simulink model "dsPIC33CK256MP508_MCLV2_QEI_Generator"  (R2022a)
settings: Solver=FixedStepDiscrete  StartTime=0.0  StopTime=12  FixedStep=.00005  RelTol=1e-3  EnableMultiTasking=on
PostLoadFcn:
  | dsPIC33CK256MP508_MCLV2_Generator_data;
InitFcn:
  | dsPIC33CK256MP508_MCLV2_Generator_data;
values from neighbouring files (symbols this model uses):
  dataType = fixdt(1,16,14)    [dsPIC33CK256MP508_MCLV2_Generator_data.m]    (also in dsPIC33CK256MP508_MCLV2_SMO_data.m; mcb_pmsm_foc_qep_dsPIC33_data.m)
  PI_params = mcb.internal.SetControllerParameters(pmsm,inverter,PU_System,T_pwm,2*Ts,Ts_speed)    [dsPIC33CK256MP508_MCLV2_Generator_data.m]    (also in dsPIC33CK256MP508_MCLV2_SMO_data.m = mcb.internal.SetControllerParameters(pmsm,inverter,PU_System; mcb_pmsm_foc_qep_dsPIC33_data.m)
  PU_System = mcb_SetPUSystem(pmsm,inverter)    [dsPIC33CK256MP508_MCLV2_Generator_data.m]    (also in dsPIC33CK256MP508_MCLV2_SMO_data.m; mcb_pmsm_foc_qep_dsPIC33_data.m)
  PWM_frequency = 20e3    (= 20000)    [dsPIC33CK256MP508_MCLV2_Generator_data.m]    (also in dsPIC33CK256MP508_MCLV2_SMO_data.m; mcb_pmsm_foc_qep_dsPIC33_data.m)
  Ts = T_pwm    (= 5e-05)    [dsPIC33CK256MP508_MCLV2_Generator_data.m]    (also in dsPIC33CK256MP508_MCLV2_SMO_data.m; mcb_pmsm_foc_qep_dsPIC33_data.m)
  Ts_speed = 10*Ts    (= 0.0005)    [dsPIC33CK256MP508_MCLV2_Generator_data.m]    (also in dsPIC33CK256MP508_MCLV2_SMO_data.m = 0.0015; mcb_pmsm_foc_qep_dsPIC33_data.m)
undefined symbols (not defined in the file or in its folder): A4, AN1, B0, B15, B2, B9, C9, D1, D2, D6, inverter, MaxPer, P20, P32, P41, P47, P57, P65, P66, P70, Pin, pmsm, PWM1max, Resol, s, us
libraries: MCHP_Blockset x14, simulink x10, mcbcontrolslib x8, slpidlib x2, mcbpositiondecoderlib x2
(part 2 of 2)

== system dsPIC33CK256MP508_MCLV2_QEI_Generator/MOTOR Cmd ==
  PWM (abc) : Inport
  Dead time Compensation : Bias  Bias=round( (2e-6/5e-5) *PWM1max )  SaturateOnIntegerOverflow=off
  Demux : Demux  Outputs=3
  PWM_HS_FEP : MCHP_Blockset/PWM IO/PWM_HS_FEP  Priority=-2000  PWMx_MODSEL=Center Aligned  PWMx_CLKSEL=no scaling  PWM_ClockResolution_DIVSEL=Dynamic Options  PWM_ClockResolution_DIVSEL_TXT=auto  PWM_ClockResolution_FSCL=Dynamic Options  PWM_ClockResolution_FSCL_TXT=auto - no jitter  PWM_ClockResolution_NoScaling=Dynamic Options  PWM_ClockResolution_NoScaling_TXT="Resol: 0.005(us)  -  MaxPer: 0.000328(s)"  MaxPeriod_s=50e-6  InitPeriode_s=50e-6  InitDutyCycleP_s=2e-6  InitDutyCycleS_s=10e-6  InitPhase_s=-1  evalin_ws=PWM1max=MCHP_Fun.Hex2num('40B3880000000000');PWM2max=MCHP_Fun.Hex2num('40B3880000000000');PWM3max=MCHP_Fun.Hex2num('40B3880000000000');  SampleTime=-1  S_INPUT=[-1]  S_INPUT_Size=[3]  S_OUTPUT=[]  S_OUTPUT_Size=[]  S_ListCustomDatatype=S.S_ListCustomDatatype={};  MCHP_USER_INTERRUPTS=0  MCHP_PORT={PWMH1 }{PWMH1}32:4:B14;{PWMH2 }{PWMH2}32:4:B12;{PWMH3 }{PWMH3}32:4:B10;{PWML1}{PWML1}32:4:B15;{PWML2}{PWML2}32:4:B13;{PWML3}{PWML3}32:4:B11;  MCHP_MASTERLINK=dsPIC33CK256MP508_MCLV2_QEI_Generator/Hardware Init/Microchip Master  MCHP_CRC=4854455  PWMx_PMOD=Complementary  PWM1_HL=PWMxH & PWMxL output enabled  PWM1_swap=off  PWM1H_pol=off  PWM1L_pol=off  PWM2_HL=PWMxH & PWMxL output enabled  PWM2_swap=off  PWM2H_pol=off  PWM2L_pol=off  PWM3_HL=PWMxH & PWMxL output enabled  PWM3_swap=off  PWM3H_pol=off  PWM3L_pol=off  PWM4_HL=not used  PWM4_swap=off  PWM4H_pol=off  PWM4L_pol=off  PWM5_HL=not used  PWM5_swap=off  PWM5H_pol=off  PWM5L_pol=off  PWM6_HL=not used  PWM6_swap=off  PWM6H_pol=off  PWM6L_pol=off  PWM7_HL=not used  PWM7_swap=off  PWM7H_pol=off  PWM7L_pol=off  PWM8_HL=not used  PWM8_swap=off  PWM8H_pol=off  PWM8L_pol=off  PWM9_HL=not used  PWM9_swap=off  PWM9H_pol=off  PWM9L_pol=off  PWM10_HL=not used  PWM10_swap=off  PWM10H_pol=off  PWM10L_pol=off  PWM11_HL=not used  PWM11_swap=off  PWM11H_pol=off  PWM11L_pol=off  PWM12_HL=not used  PWM12_swap=off  PWM12H_pol=off  PWM12L_pol=off  PWM1_ShowTrig=on  PWM1_Init_PGxTRIGABC_s=[0 -1 -1 ]  PWM1_ADTRxEN1=ADC Trigger 1  PWM1_ADTRxEN2=none  PWM1_ADTRxEN3=none  PWM2_ShowTrig=off  PWM2_Init_PGxTRIGABC_s=[-1 -1 -1]  PWM2_ADTRxEN1=none  PWM2_ADTRxEN2=none  PWM2_ADTRxEN3=none  PWM3_ShowTrig=off  PWM3_Init_PGxTRIGABC_s=[-1 -1 -1]  PWM3_ADTRxEN1=none  PWM3_ADTRxEN2=none  PWM3_ADTRxEN3=none  PWM4_ShowTrig=off  PWM4_Init_PGxTRIGABC_s=[-1 -1 -1]  PWM4_ADTRxEN1=none  PWM4_ADTRxEN2=none  PWM4_ADTRxEN3=none  PWM5_ShowTrig=off  PWM5_Init_PGxTRIGABC_s=[-1 -1 -1]  PWM5_ADTRxEN1=none  PWM5_ADTRxEN2=none  PWM5_ADTRxEN3=none  PWM6_ShowTrig=off  PWM6_Init_PGxTRIGABC_s=[-1 -1 -1]  PWM6_ADTRxEN1=none  PWM6_ADTRxEN2=none  PWM6_ADTRxEN3=none  PWM7_ShowTrig=off  PWM7_Init_PGxTRIGABC_s=[-1 -1 -1]  PWM7_ADTRxEN1=none  PWM7_ADTRxEN2=none  PWM7_ADTRxEN3=none  PWM8_ShowTrig=off  PWM8_Init_PGxTRIGABC_s=[-1 -1 -1]  PWM8_ADTRxEN1=none  PWM8_ADTRxEN2=none  PWM8_ADTRxEN3=none  BlockInput_VectorScalar=Independant Scalar  BlockInput_Period=Not a block input  BlockInput_DutyCycle=a Uint raw input (PWMxmax variable represent max period)  BlockInput_PhaseShift=Not a block input  BlockInput_SEVTCMP=Not a block input  BlockInput_TRIGx=Not a block input  BlockInput_DeadTime=Not a block input  BlockOutput_FaultDisabled=off  BlockOutput_Fault=on  DTC=Positive dead time (ensure period of time with PWM_H and PWM_L disasserted)  FLTSRC1_DTCMP=Dynamic Options  FLTSRC1_DTCMP_TXT=<empty>  FLTSRC2_DTCMP=Dynamic Options  FLTSRC2_DTCMP_TXT=<empty>  FLTSRC3_DTCMP=Dynamic Options  FLTSRC3_DTCMP_TXT=<empty>  FLTSRC4_DTCMP=Dynamic Options  FLTSRC4_DTCMP_TXT=<empty>  FLTSRC5_DTCMP=Dynamic Options  FLTSRC5_DTCMP_TXT=<empty>  FLTSRC6_DTCMP=Dynamic Options  FLTSRC6_DTCMP_TXT=<empty>  FLTSRC7_DTCMP=Dynamic Options  FLTSRC7_DTCMP_TXT=<empty>  FLTSRC8_DTCMP=Dynamic Options  FLTSRC8_DTCMP_TXT=<empty>  FLTSRC9_DTCMP=Dynamic Options  FLTSRC9_DTCMP_TXT=<empty>  FLTSRC10_DTCMP=Dynamic Options  FLTSRC10_DTCMP_TXT=<empty>  FLTSRC11_DTCMP=Dynamic Options  FLTSRC11_DTCMP_TXT=<empty>  FLTSRC12_DTCMP=Dynamic Options  FLTSRC12_DTCMP_TXT=<empty>  DeadTime_s=1e-6  DeadTimeAlt_s=1e-6  DeadTimeComp_s=0  FLTMODx=Disabled  FLTSRCx=Dynamic Options  FLTSRCx_TXT=<empty>  FLTDATx=PWM H/L -> 11  CLMODx=Disabled  CLSRCx=Dynamic Options  CLSRCx_TXT=<empty>  CLDATx=PWM H/L -> 00  FLTLEBENx=off  CLLEBENx=off  LeadEdgeBlkPer_s=5e-7  PHRx=off  PHFx=off  PLRx=off  PLFx=off
      settings: SourceProductName=MPLAB Device Blocks for Simulink
  Saturation low side turn on errate workaround + errata for Phase shift (times 2) : Saturate  UpperLimit=PWM1max  LowerLimit=round( (2e-6/5e-5) *PWM1max )* 2
  int to uint : DataTypeConversion  OutDataTypeStr=uint16  ConvertRealWorld=Stored Integer (SI)  SaturateOnIntegerOverflow=off  RndMeth=Floor
  wires:
  int to uint/1 -> Saturation low side turn on errate workaround + errata for Phase shift (times 2)/1
  Dead time Compensation/1 -> int to uint/1
  PWM (abc)/1 -> Dead time Compensation/1
  Saturation low side turn on errate workaround + errata for Phase shift (times 2)/1 -> Demux/1
  Demux/2 -> PWM_HS_FEP/2
  Demux/3 -> PWM_HS_FEP/3
  Demux/1 -> PWM_HS_FEP/1

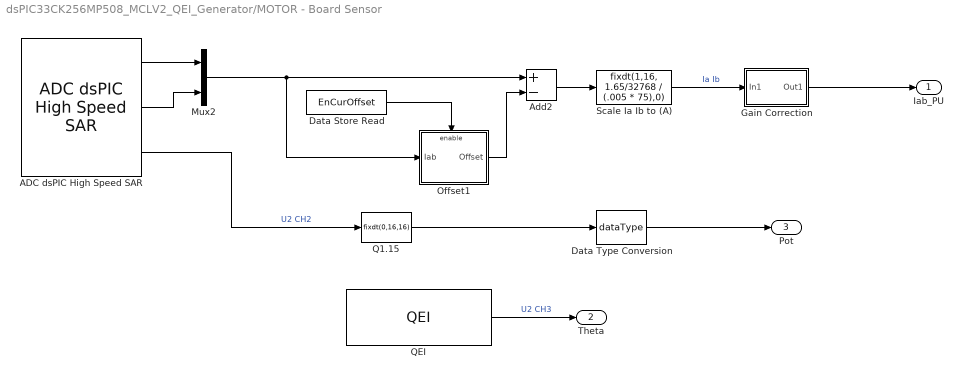
== system dsPIC33CK256MP508_MCLV2_QEI_Generator/MOTOR - Board Sensor ==
  ADC dsPIC High Speed SAR : MCHP_Blockset/Analog IO/ADC dsPIC High Speed SAR  ACLKCON=Not used  ADC_FRACT=Fractional (left aligned)  ADC_NRE=off  DMA_Size=Single trigger - (default)  ADC_Synchronisation=Triggered by custom source  ADC_Trig=Dynamic Options  ADC_Trig_TXT=PWM1 Trigger 1  ADC_TrigTimeStep=Trig model step after all sample from this block are converted  ADC_TrigInfo=0  SampleTime=Ts  S_INPUT=[]  S_INPUT_Size=[]  S_OUTPUT="[5  5]"  S_OUTPUT_Size="[1  1]"  S_ListCustomDatatype=S.S_ListCustomDatatype={};  MCHP_USER_INTERRUPTS={ADCAN1}{ADCBUF1}{ADC Data 1 Ready}{VectorName(ADCAN1Interrupt) Priority(-1) RegisterReadClear(ADCBUF1)Config_BitSet(ADIELbits.IE1) };{ADCAN3}{ADCBUF3}{ADC Data 3 Ready}{VectorName(ADCAN3Interrupt) Priority(-1) RegisterReadClear(ADCBUF3)Config_BitSet(ADIELbits.IE3) };{ADCAN18}{ADCBUF18}{ADC Data 18 Ready}{VectorName(ADCAN18Interrupt) Priority(-1) RegisterReadClear(ADCBUF18)Config_BitSet(ADIEHbits.IE18) };  MCHP_PORT={Analog Input 1}{AN1}15:2:B2;{Analog Input 4}{AN4}15:2:A4;{Analog Input 19}{AN19}15:2:D11;  MCHP_MASTERLINK=dsPIC33CK256MP508_MCLV2_QEI_Generator/Hardware Init/Microchip Master  MCHP_CRC=4029738  ADC_Info=Total Time = 4.92(us)  ADC0_pin=Dynamic Options  ADC0_pin_TXT=Not used  ADC0_R="< 50   kOhm"  ADC0_res=12 bits  ADC0_signed=signed 16 bits  ADC0_FILTER=No Oversampling  ADC0_FILTER_nSamples=256 samples  ADC0_STRGEN=Start sampling followed by conversion  ADC0_STRGEN_on=Start sampling followed by conversion  ADC0_SSAMPEN=off  ADC0_Info=tSmp_min=20(ns) x 0 = 0(s) ; tConv=210(ns) x 0 = 0(s) ; TOTAL=0(s)  ADC1_pin=Dynamic Options  ADC1_pin_TXT=AN1 / B2 / Pin[41]  ADC1_R="< 50   kOhm"  ADC1_res=12 bits  ADC1_signed=signed 16 bits  ADC1_FILTER=No Oversampling  ADC1_FILTER_nSamples=128 samples  ADC1_STRGEN=Start sampling followed by conversion  ADC1_STRGEN_on=Start sampling followed by conversion  ADC1_SSAMPEN=off  ADC1_Info=tSmp_min=2.06(us) x 1 = 2.06(us) ; tConv=370(ns) x 1 = 370(ns) ; TOTAL=2.44(us)  ADC2_pin=Dynamic Options  ADC2_pin_TXT=Not used  ADC2_R="< 5    kOhm"  ADC2_res=12 bits  ADC2_signed=signed 16 bits  ADC2_FILTER=No Oversampling  ADC2_FILTER_nSamples=256 samples  ADC2_STRGEN=End sampling and start conversion  ADC2_STRGEN_on=Start sampling followed by conversion  ADC2_SSAMPEN=on  ADC2_Info=tSmp_min=14.706(ns) x 0 = 0(s) ; tConv=154.41(ns) x 0 = 0(s) ; TOTAL=0(s)  ADC3_pin=Dynamic Options  ADC3_pin_TXT=Not used  ADC3_R="< 10   kOhm"  ADC3_res=12 bits  ADC3_signed=signed 16 bits  ADC3_FILTER=Burst convert of n samples are Summed  ADC3_FILTER_nSamples=64 samples  ADC3_STRGEN=End sampling and start conversion  ADC3_STRGEN_on=Start sampling followed by conversion  ADC3_SSAMPEN=on  ADC3_Info=tSmp_min=14.706(ns) x 0 = 0(s) ; tConv=154.41(ns) x 0 = 0(s) ; TOTAL=0(s)  ADC4_pin=Dynamic Options  ADC4_pin_TXT=Not used  ADC4_R=< 200 Ohm  ADC4_res=12 bits  ADC4_signed=unsigned 16 bits  ADC4_FILTER=No Oversampling  ADC4_FILTER_nSamples=256 samples  ADC4_STRGEN=End sampling and start conversion  ADC4_STRGEN_on=Start sampling followed by conversion  ADC4_SSAMPEN=off  ADC4_Info=tSmp_min=14.706(ns) x 0 = 0(s) ; tConv=154.41(ns) x 0 = 0(s) ; TOTAL=0(s)  ADC5_pin=Dynamic Options  ADC5_pin_TXT=Not used  ADC5_R=< 200 Ohm  ADC5_res=12 bits  ADC5_signed=unsigned 16 bits  ADC5_FILTER=Burst convert of n samples are Summed  ADC5_FILTER_nSamples=256 samples  ADC5_STRGEN=End sampling and start conversion  ADC5_STRGEN_on=Start sampling followed by conversion  ADC5_SSAMPEN=on  ADC5_Info=tSmp_min=14.706(ns) x 0 = 0(s) ; tConv=154.41(ns) x 0 = 0(s) ; TOTAL=0(s)  ADC6_pin=Dynamic Options  ADC6_pin_TXT=Not used  ADC6_R=< 200 Ohm  ADC6_res=12 bits  ADC6_signed=unsigned 16 bits  ADC6_FILTER=Burst convert of n samples are Summed  ADC6_FILTER_nSamples=256 samples  ADC6_STRGEN=End sampling and start conversion  ADC6_STRGEN_on=Start sampling followed by conversion  ADC6_SSAMPEN=on  ADC6_Info=tSmp_min=14.706(ns) x 0 = 0(s) ; tConv=154.41(ns) x 0 = 0(s) ; TOTAL=0(s)  ADC7_R="< 50   kOhm"  ADC7_res=12 bits  ADC7_AN0=Not used  ADC7_AN1=Not used  ADC7_AN2=Not used  ADC7_AN3=Not used  ADC7_AN4=signed int16  ADC7_AN5=Not used  ADC7_AN6=Not used  ADC7_AN7=Not used  ADC7_AN8=Not used  ADC7_AN9=Not used  ADC7_AN10=Not used  ADC7_AN11=Not used  ADC7_AN12=Not used  ADC7_AN13=Not used  ADC7_AN14=Not used  ADC7_AN15=Not used  ADC7_AN16=Not used  ADC7_AN17=Not used  ADC7_AN18=Not used  ADC7_AN19=unsigned int16  ADC7_AN20=Not used  ADC7_AN21=Not used  ADC7_AN22=Not used  ADC7_AN23=Not used  ADC7_AN24=Not used  ADC7_AN25=Not used  ADC7_AN26=Not used  ADC7_AN27=Not used  ADC7_AN28=Not used  ADC7_AN29=Not used  ADC7_AN30=Not used  ADC7_AN31=Not used  IVref=Not used  IVTemp=Not used  ADC7_Info=tSmp_min=2.08(us) x 2 = 4.16(us) ; tConv=370(ns) x 2 = 740(ns) ; TOTAL=4.92(us)
      settings: SourceProductName=MPLAB Device Blocks for Simulink
  Add2 : Sum  Inputs=+-  OutDataTypeStr=int16  RndMeth=Simplest
  Data Store Read : DataStoreRead  DataStoreName=EnCurOffset  IndexOptions=Index vector (dialog)  Indices=1  OutputSizes=1
  Data Type Conversion : DataTypeConversion  OutDataTypeStr=dataType  RndMeth=Simplest  SaturateOnIntegerOverflow=off
  Gain Correction : Subsystem
  Mux2 : Mux  Inputs=2
  Offset1 : Subsystem
  Q1.15 : DataTypeConversion  OutDataTypeStr=fixdt(0,16,16)  ConvertRealWorld=Stored Integer (SI)  SaturateOnIntegerOverflow=off  RndMeth=Floor
  QEI : MCHP_Blockset/QEI/QEI  QEI_REF=1  QEI_MODE=Quadrature Encoder  QEI_x2mode=off  QEI_PulseCountDir=Down  PIN_QEA=Dynamic Options  PIN_QEA_TXT=D1 / P65 / Pin[73]  PIN_QEB=Dynamic Options  PIN_QEB_TXT=D2 / P66 / Pin[72]  SWPAB=on  QEAPOL=off  QEBPOL=off  SampleTime=Ts  PIN_CCMP=Dynamic Options  PIN_CCMP_TXT=A4 / P20 / Pin[33]  MCHP_PORT={QEI1 A}{QEIA1}5:0:P65;{QEI1 B}{QEIB1}5:0:P66;  MCHP_MASTERLINK=dsPIC33CK256MP508_MCLV2_QEI_Generator/Hardware Init/Microchip Master  INDXxCNT_Output=is not an output  POSxCNT_Output=is a 16 bits unsigned block output  RESET_Input=off  PIMOD_mode=position is cyclique between user defined boundaries  PIMOD_modeB=Never reset position  PIMOD_reset=on next INDEX event  PIN_INDEX=Dynamic Options  PIN_INDEX_TXT=B15 / P47 / Pin[3]  IMV=QEA = 1 and QEB = 0  IMV_x2=QEA = 1  PIN_HOME=Dynamic Options  PIN_HOME_TXT=B9 / P41 / Pin[61]  QEIxLEC_GEC=[0 999]  QEIxIC=0  PCIIRQ=off  IDXPOL=off  HOMPOL=on  VELxCNT_Output=is not an output  INTxHLD_Output=is not an output  MaxPeriod=0.1  FILTREN=on  QFDIV_popup=Dynamic Options  QFDIV_popup_TXT=520.83 kHz  FILTER_CutOffFreq=100e3  QEI_IntPri=5
      settings: SourceProductName=MPLAB Device Blocks for Simulink
  Scale Ia Ib to (A) : DataTypeConversion  OutDataTypeStr=fixdt(1,16, 1.65/32768 / (.005 * 75),0)  ConvertRealWorld=Stored Integer (SI)  SaturateOnIntegerOverflow=off  RndMeth=Floor
  Iab_PU : Outport  VectorParamsAs1DForOutWhenUnconnected=off
  Theta : Outport  Port=2  VectorParamsAs1DForOutWhenUnconnected=off
  Pot : Outport  Port=3  VectorParamsAs1DForOutWhenUnconnected=off
  wires:
  QEI/1 -> Theta/1  "U2 CH3"
  Mux2/1 -> Add2/1, Offset1/1(Iab)
  ADC dsPIC High Speed SAR/3 -> Q1.15/1  "U2 CH2"
  Q1.15/1 -> Data Type Conversion/1
  Scale Ia Ib to (A)/1 -> Gain Correction/1(In1)  "Ia Ib"
  Offset1/1(Offset) -> Add2/2
  Add2/1 -> Scale Ia Ib to (A)/1
  Data Store Read/1 -> Offset1/Enable
  Data Type Conversion/1 -> Pot/1
  Gain Correction/1(Out1) -> Iab_PU/1
  ADC dsPIC High Speed SAR/1 -> Mux2/1
  ADC dsPIC High Speed SAR/2 -> Mux2/2

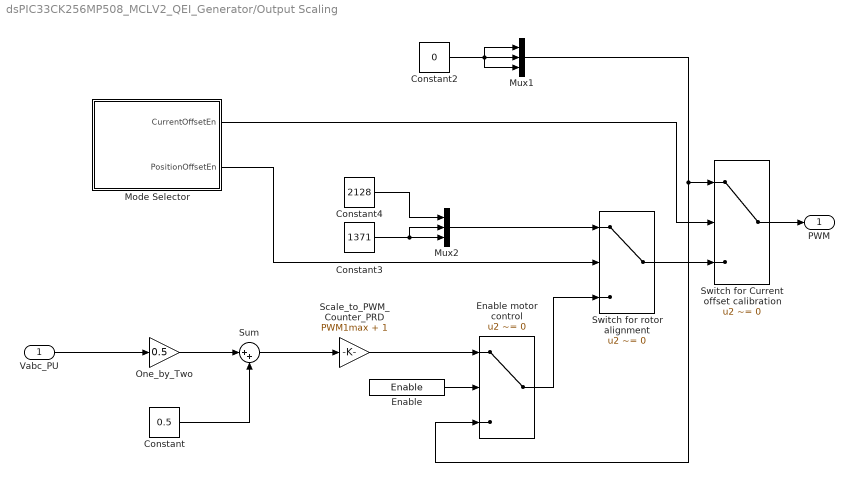
== system dsPIC33CK256MP508_MCLV2_QEI_Generator/Output Scaling ==
  Vabc_PU : Inport
  Constant : Constant  Value=0.5  OutDataTypeStr=dataType  SampleTime=-1
  Constant2 : Constant  Value=0  OutDataTypeStr=Inherit: Inherit via back propagation
  Constant3 : Constant  Value=1371  OutDataTypeStr=Inherit: Inherit via back propagation
  Constant4 : Constant  Value=2128  OutDataTypeStr=Inherit: Inherit via back propagation
  Enable : DataStoreRead  DataStoreName=Enable  IndexOptions=Index vector (dialog)  Indices=1  OutputSizes=1
  Enable motor control : Switch  Criteria=u2 ~= 0  Threshold=250  SaturateOnIntegerOverflow=off  InputSameDT=off
  Mode Selector : Subsystem
  Mux1 : Mux  Inputs=3
  Mux2 : Mux  Inputs=3
  One_by_Two : Gain  Gain=0.5  RndMeth=Simplest  OutDataTypeStr=Inherit: Same as input
  Scale_to_PWM_Counter_PRD : Gain  Gain=PWM1max + 1  OutDataTypeStr=uint16  RndMeth=Simplest
  Sum : Sum  Inputs=|++
  Switch for Current offset calibration : Switch  Criteria=u2 ~= 0  Threshold=250  SaturateOnIntegerOverflow=off  InputSameDT=off
  Switch for rotor alignment : Switch  Criteria=u2 ~= 0  Threshold=250  SaturateOnIntegerOverflow=off  InputSameDT=off
  PWM : Outport
  wires:
  Sum/1 -> Scale_to_PWM_Counter_PRD/1
  Constant/1 -> Sum/2
  Switch for Current offset calibration/1 -> PWM/1
  One_by_Two/1 -> Sum/1
  Switch for rotor alignment/1 -> Switch for Current offset calibration/3
  Scale_to_PWM_Counter_PRD/1 -> Enable motor control/1
  Vabc_PU/1 -> One_by_Two/1
  Mode Selector/2(PositionOffsetEn) -> Switch for rotor alignment/2
  Mux2/1 -> Switch for rotor alignment/1
  Mux1/1 -> Enable motor control/3, Switch for Current offset calibration/1
  Constant2/1 -> Mux1/1, Mux1/3, Mux1/2
  Constant3/1 -> Mux2/3, Mux2/2
  Constant4/1 -> Mux2/1
  Mode Selector/1(CurrentOffsetEn) -> Switch for Current offset calibration/2
  Enable/1 -> Enable motor control/2
  Enable motor control/1 -> Switch for rotor alignment/3

== system dsPIC33CK256MP508_MCLV2_QEI_Generator/Serial Tx ==
  Data : Inport
  Counter Limited : simulink/Sources/Counter Limited  uplimit=3  tsamp=-1
  Data Type Conversion : DataTypeConversion  OutDataTypeStr=uint8  RndMeth=Simplest  SaturateOnIntegerOverflow=off
  Demux : Demux
  Index Vector : MultiPortSwitch  DataPortOrder=Zero-based contiguous  Inputs=4  zeroidx=on  OutDataTypeStr=Inherit: Same as first data input  RndMeth=Simplest  SaturateOnIntegerOverflow=off  InputSameDT=off
  UART_TX : Subsystem
  wires:
  Data Type Conversion/1 -> UART_TX/1(Count), Index Vector/1
  Index Vector/1 -> UART_TX/2(Data)
  Demux/4 -> Index Vector/5
  Demux/3 -> Index Vector/4
  Demux/1 -> Index Vector/2
  Demux/2 -> Index Vector/3
  Data/1 -> Demux/1
  Counter Limited/1 -> Data Type Conversion/1

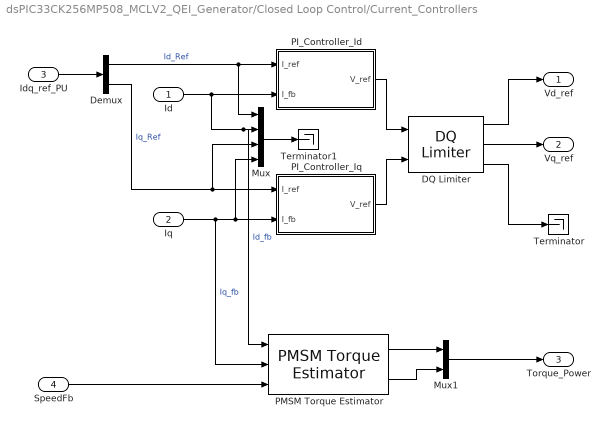
== system dsPIC33CK256MP508_MCLV2_QEI_Generator/Closed Loop Control/Current_Controllers ==
  Id : Inport
  Iq : Inport  Port=2
  Idq_ref_PU : Inport  Port=3
  SpeedFb : Inport  Port=4
  DQ Limiter : mcbcontrolslib/DQ Limiter  Vmax=0.95
      settings: SourceProductBaseCode=MT
  Demux : Demux  Outputs=2
  Mux : Mux
  Mux1 : Mux  Inputs=2
  PI_Controller_Id : Subsystem
  PI_Controller_Iq : Subsystem
  PMSM Torque Estimator : mcbcontrolslib/PMSM Torque Estimator  polePairs=pmsm.p  Ld=pmsm.Ld  Lq=pmsm.Lq  FluxPM=pmsm.FluxPM  Units=Per-Unit (PU)  V_base=PU_System.V_base  I_base=PU_System.I_base  N_base=PU_System.N_base  T_base=0.26345  P_base=91.4523
      settings: SourceProductBaseCode=MT
  Terminator : Terminator
  Terminator1 : Terminator
  Vd_ref : Outport  VectorParamsAs1DForOutWhenUnconnected=off
  Vq_ref : Outport  Port=2  VectorParamsAs1DForOutWhenUnconnected=off
  Torque_Power : Outport  Port=3  VectorParamsAs1DForOutWhenUnconnected=off
  wires:
  Iq/1 -> PMSM Torque Estimator/2, Mux/4, PI_Controller_Iq/2(I_fb)  "Iq_fb"
  Id/1 -> PMSM Torque Estimator/1, Mux/2, PI_Controller_Id/2(I_fb)  "Id_fb"
  Demux/1 -> Mux/1, PI_Controller_Id/1(I_ref)  "Id_Ref"
  Demux/2 -> Mux/3, PI_Controller_Iq/1(I_ref)  "Iq_Ref"
  Idq_ref_PU/1 -> Demux/1
  PI_Controller_Id/1(V_ref) -> DQ Limiter/1
  PI_Controller_Iq/1(V_ref) -> DQ Limiter/2
  DQ Limiter/1 -> Vd_ref/1
  DQ Limiter/2 -> Vq_ref/1
  DQ Limiter/3 -> Terminator/1
  Mux/1 -> Terminator1/1
  SpeedFb/1 -> PMSM Torque Estimator/3
  PMSM Torque Estimator/1 -> Mux1/1
  PMSM Torque Estimator/2 -> Mux1/2
  Mux1/1 -> Torque_Power/1

== system dsPIC33CK256MP508_MCLV2_QEI_Generator/Hardware Init/Enable Switch ==
  Codegen : Subsystem  VariantControl=(codegen)
  Sim : Subsystem  VariantControl=(sim)

== system dsPIC33CK256MP508_MCLV2_QEI_Generator/Hardware Init/Open Board and Motor pages ==

== system dsPIC33CK256MP508_MCLV2_QEI_Generator/Input Scaling/Position Offset ==
  Iab : Inport
  Enable : EnablePort
  Offset : Outport
  wires:
  Iab/1 -> Offset/1

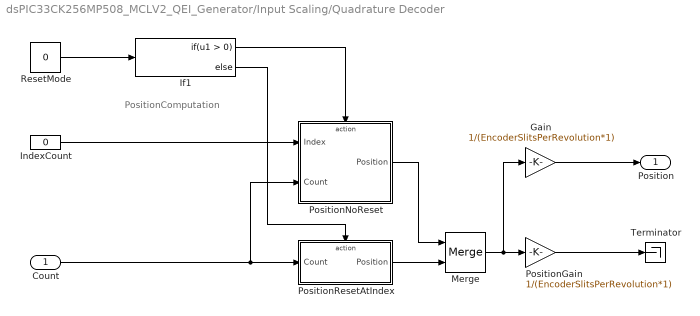
== system dsPIC33CK256MP508_MCLV2_QEI_Generator/Input Scaling/Quadrature Decoder ==
  note: PositionComputation
  Count : Inport  OutDataTypeStr=uint16
  Gain : Gain  Gain=1/(EncoderSlitsPerRevolution*1)  ParamDataTypeStr=fixdt(0,16)  OutDataTypeStr=PositionDataType  RndMeth=Simplest
  If1 : If
  IndexCount : Constant  Value=0  OutDataTypeStr=uint16
  Merge : Merge
  PositionGain : Gain  Gain=1/(EncoderSlitsPerRevolution*1)  ParamDataTypeStr=fixdt(0,16)  OutDataTypeStr=PositionDataType  RndMeth=Simplest
  PositionNoReset : Subsystem
  PositionResetAtIndex : Subsystem  TreatAsAtomicUnit=on
  ResetMode : Constant  Value=0  OutDataTypeStr=int16
  Terminator : Terminator
  Position : Outport  VectorParamsAs1DForOutWhenUnconnected=off
  wires:
  If1/1 -> PositionNoReset/Action
  PositionNoReset/1(Position) -> Merge/1
  Merge/1 -> Gain/1, PositionGain/1
  If1/2 -> PositionResetAtIndex/Action
  PositionResetAtIndex/1(Position) -> Merge/2
  Count/1 -> PositionResetAtIndex/1(Count), PositionNoReset/2(Count)
  ResetMode/1 -> If1/1
  IndexCount/1 -> PositionNoReset/1(Index)
  PositionGain/1 -> Terminator/1
  Gain/1 -> Position/1

== system dsPIC33CK256MP508_MCLV2_QEI_Generator/MOTOR - Board Sensor/Gain Correction ==
  In1 : Inport
  Demux : Demux  Outputs=2
  Gain : Gain  Gain=0.865  RndMeth=Zero  OutDataTypeStr=Inherit: Same as input
  Gain1 : Gain  Gain=0.961  RndMeth=Zero  OutDataTypeStr=Inherit: Same as input
  Mux : Mux  Inputs=2
  To Per-Unit : Gain  Gain=inverter.invertingAmp/PU_System.I_base  OutMin=-1  OutMax=1  OutDataTypeStr=fixdt(1,16)  RndMeth=Zero
  Out1 : Outport
  wires:
  Demux/1 -> Gain/1
  To Per-Unit/1 -> Demux/1
  Gain/1 -> Mux/1
  Mux/1 -> Out1/1
  In1/1 -> To Per-Unit/1
  Demux/2 -> Gain1/1
  Gain1/1 -> Mux/2

== system dsPIC33CK256MP508_MCLV2_QEI_Generator/MOTOR - Board Sensor/Offset1 ==
  Iab : Inport
  Enable : EnablePort
  Offset : Outport
  wires:
  Iab/1 -> Offset/1

== system dsPIC33CK256MP508_MCLV2_QEI_Generator/Output Scaling/Mode Selector ==
  Delay : Delay  DelayLength=1
  NOT : Logic  Operator=NOT  IconShape=distinctive  AllPortsSameDT=off  OutDataTypeStr=boolean
  Subsystem1 : Subsystem
  Up Counter : Subsystem
  CurrentOffsetEn : Outport
  PositionOffsetEn : Outport  Port=2
  wires:
  Up Counter/1(Count) -> Subsystem1/1(Count)
  Delay/1 -> NOT/1
  NOT/1 -> Up Counter/Enable
  Subsystem1/3(EnClosedLoop) -> Delay/1
  Subsystem1/1(Current Offset) -> CurrentOffsetEn/1
  Subsystem1/2(PositionOffset) -> PositionOffsetEn/1

== system dsPIC33CK256MP508_MCLV2_QEI_Generator/Serial Tx/UART_TX ==
  Count : Inport
  Data : Inport  Port=2
  Debug_Data : Subsystem
  SCI_Tx : Subsystem
  wires:
  Count/1 -> Debug_Data/1(Count)
  Debug_Data/1(Data_log) -> SCI_Tx/1(Data_Log)
  Data/1 -> Debug_Data/2(Data)

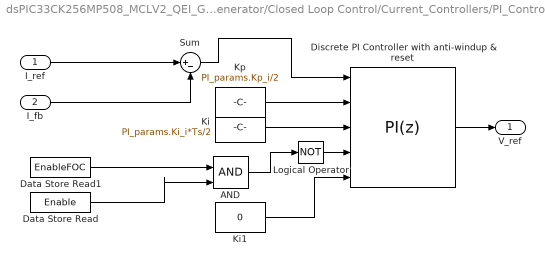
== system dsPIC33CK256MP508_MCLV2_QEI_Generator/Closed Loop Control/Current_Controllers/PI_Controller_Id ==
  I_ref : Inport
  I_fb : Inport  Port=2
  AND : Logic  IconShape=distinctive  AllPortsSameDT=off  OutDataTypeStr=boolean
  Data Store Read : DataStoreRead  DataStoreName=Enable  IndexOptions=Index vector (dialog)  Indices=1  OutputSizes=1
  Data Store Read1 : DataStoreRead  DataStoreName=EnableFOC  IndexOptions=Index vector (dialog)  Indices=1  OutputSizes=1
  Discrete PI Controller with anti-windup & reset : slpidlib/PID Controller  Controller=PI  Form=Parallel  TimeDomain=Discrete-time  UseExternalTs=off  SampleTime=-1  IntegratorMethod=Forward Euler  FilterMethod=Forward Euler  ControllerParametersSource=external  P=1  I=1  UseKiTs=on  D=0  N=100  UseFilter=on  TunerSelectOption=Transfer Function Based (PID Tuner App)  InitialConditionSource=external  InitialConditionForIntegrator=0  InitialConditionForFilter=0  DifferentiatorICPrevScaledInput=0  ExternalReset=level  TrackingMode=off  Kt=1  LimitOutput=on  SatLimitsSource=internal  UpperSaturationLimit=1  LowerSaturationLimit=-1  LinearizeAsGain=on  AntiWindupMode=clamping  Kb=1  RndMeth=Simplest  POutMin=[]  POutMax=[]  IOutMin=[]  IOutMax=[]  DOutMin=[]  DOutMax=[]  NOutMin=[]  NOutMax=[]  SumOutMin=[]  SumOutMax=[]  SaturationOutDataTypeStr=Inherit: Inherit via back propagation  SaturationOutMin=[]  SaturationOutMax=[]  PParamMin=[]  PParamMax=[]  IParamMin=[]  IParamMax=[]  DParamMin=[]  DParamMax=[]  NParamMin=[]  NParamMax=[]  KbParamMin=[]  KbParamMax=[]  KtParamMin=[]  KtParamMax=[]  KbOutMin=[]  KbOutMax=[]  KtOutMin=[]  KtOutMax=[]  IntegratorOutMin=[]  IntegratorOutMax=[]  FilterOutMin=[]  FilterOutMax=[]  SumI1OutMin=[]  SumI1OutMax=[]  SumI2OutMin=[]  SumI2OutMax=[]  SumI3OutMin=[]  SumI3OutMax=[]  SumI4OutMin=[]  SumI4OutMax=[]  SumDOutMin=[]  SumDOutMax=[]  DifferentiatorOutMin=[]  DifferentiatorOutMax=[]  FilterDiffOutCoefMin=[]  FilterDiffOutCoefMax=[]  ReciprocalOutMin=[]  ReciprocalOutMax=[]  SumDenOutMin=[]  SumDenOutMax=[]  SumNumOutMin=[]  SumNumOutMax=[]  DivideOutMin=[]  DivideOutMax=[]  UdiffTsProdOutMin=[]  UdiffTsProdOutMax=[]  NTsProdOutMin=[]  NTsProdOutMax=[]  UintegralTsProdOutMin=[]  UintegralTsProdOutMax=[]  UngainTsProdOutMin=[]  UngainTsProdOutMax=[]  IntegratorContinuousStateAttributes=''  IntegratorStateMustResolveToSignalObject=off  IntegratorRTWStateStorageClass=Auto  FilterContinuousStateAttributes=''  FilterStateMustResolveToSignalObject=off  FilterRTWStateStorageClass=Auto  ParallelPVariant=ExternalParameters  IdealPVariant=Disabled  IVariant=ExternalParameters  DVariant=Disabled  IntegratorVariant=Discrete  SatVariant=Enabled  AWVariant=DiscClampingParallel  PCopyVariant=Disabled  TRVariant=Disabled  FdbkBlocksVariant=Forward  IdealPFdbkVariant=Disabled  SatFdbkVariant=Disabled  DerivativeFilterVariant=Disabled  NVariant=Disabled  NCopyVariant=Disabled_SignalSpec  FilterICVariant=Disabled  IntegratorICVariant=ExternalICs  ExternalResetVariant=ExternalReset  TRSumVariant=Passthrough  SumFdbkVariant=Disabled  SumVariant=Sum_PI  TsampFilterVariant=InternalTs  TsampNgainVariant=Passthrough  TsampIntegralVariant=Passthrough  ExternalSaturationOutDataTypeStr=Inherit: Same as second input  aMode=5
  Ki : Constant  Value=PI_params.Ki_i*Ts/2  OutDataTypeStr=dataType  SampleTime=-1
  Ki1 : Constant  Value=0  OutDataTypeStr=dataType  SampleTime=-1
  Kp : Constant  Value=PI_params.Kp_i/2  OutDataTypeStr=dataType2  SampleTime=-1
  Logical Operator : Logic  Operator=NOT  IconShape=distinctive  AllPortsSameDT=off  OutDataTypeStr=boolean
  Sum : Sum  Inputs=|+-  OutDataTypeStr=Inherit: Same as first input
  V_ref : Outport  VectorParamsAs1DForOutWhenUnconnected=off
  wires:
  I_ref/1 -> Sum/1
  I_fb/1 -> Sum/2
  Data Store Read1/1 -> AND/1
  Discrete PI Controller with anti-windup & reset/1 -> V_ref/1
  Sum/1 -> Discrete PI Controller with anti-windup & reset/1
  Kp/1 -> Discrete PI Controller with anti-windup & reset/2
  Ki/1 -> Discrete PI Controller with anti-windup & reset/3
  Logical Operator/1 -> Discrete PI Controller with anti-windup & reset/4
  Ki1/1 -> Discrete PI Controller with anti-windup & reset/5
  Data Store Read/1 -> AND/2
  AND/1 -> Logical Operator/1

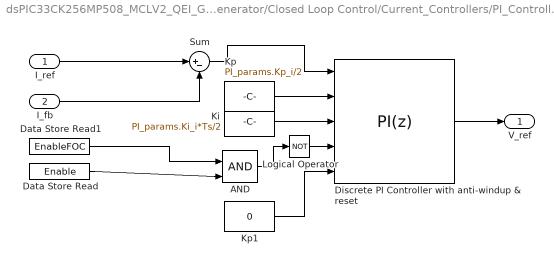
== system dsPIC33CK256MP508_MCLV2_QEI_Generator/Closed Loop Control/Current_Controllers/PI_Controller_Iq ==
  I_ref : Inport
  I_fb : Inport  Port=2
  AND : Logic  IconShape=distinctive  AllPortsSameDT=off  OutDataTypeStr=boolean
  Data Store Read : DataStoreRead  DataStoreName=Enable  IndexOptions=Index vector (dialog)  Indices=1  OutputSizes=1
  Data Store Read1 : DataStoreRead  DataStoreName=EnableFOC  IndexOptions=Index vector (dialog)  Indices=1  OutputSizes=1
  Discrete PI Controller with anti-windup & reset : slpidlib/PID Controller  Controller=PI  Form=Parallel  TimeDomain=Discrete-time  UseExternalTs=off  SampleTime=-1  IntegratorMethod=Forward Euler  FilterMethod=Forward Euler  ControllerParametersSource=external  P=1  I=1  UseKiTs=on  D=0  N=100  UseFilter=on  TunerSelectOption=Transfer Function Based (PID Tuner App)  InitialConditionSource=external  InitialConditionForIntegrator=0  InitialConditionForFilter=0  DifferentiatorICPrevScaledInput=0  ExternalReset=level  TrackingMode=off  Kt=1  LimitOutput=on  SatLimitsSource=internal  UpperSaturationLimit=1  LowerSaturationLimit=-1  LinearizeAsGain=on  AntiWindupMode=clamping  Kb=1  RndMeth=Simplest  POutMin=[]  POutMax=[]  IOutMin=[]  IOutMax=[]  DOutMin=[]  DOutMax=[]  NOutMin=[]  NOutMax=[]  SumOutMin=[]  SumOutMax=[]  SaturationOutDataTypeStr=Inherit: Inherit via back propagation  SaturationOutMin=[]  SaturationOutMax=[]  PParamMin=[]  PParamMax=[]  IParamMin=[]  IParamMax=[]  DParamMin=[]  DParamMax=[]  NParamMin=[]  NParamMax=[]  KbParamMin=[]  KbParamMax=[]  KtParamMin=[]  KtParamMax=[]  KbOutMin=[]  KbOutMax=[]  KtOutMin=[]  KtOutMax=[]  IntegratorOutMin=[]  IntegratorOutMax=[]  FilterOutMin=[]  FilterOutMax=[]  SumI1OutMin=[]  SumI1OutMax=[]  SumI2OutMin=[]  SumI2OutMax=[]  SumI3OutMin=[]  SumI3OutMax=[]  SumI4OutMin=[]  SumI4OutMax=[]  SumDOutMin=[]  SumDOutMax=[]  DifferentiatorOutMin=[]  DifferentiatorOutMax=[]  FilterDiffOutCoefMin=[]  FilterDiffOutCoefMax=[]  ReciprocalOutMin=[]  ReciprocalOutMax=[]  SumDenOutMin=[]  SumDenOutMax=[]  SumNumOutMin=[]  SumNumOutMax=[]  DivideOutMin=[]  DivideOutMax=[]  UdiffTsProdOutMin=[]  UdiffTsProdOutMax=[]  NTsProdOutMin=[]  NTsProdOutMax=[]  UintegralTsProdOutMin=[]  UintegralTsProdOutMax=[]  UngainTsProdOutMin=[]  UngainTsProdOutMax=[]  IntegratorContinuousStateAttributes=''  IntegratorStateMustResolveToSignalObject=off  IntegratorRTWStateStorageClass=Auto  FilterContinuousStateAttributes=''  FilterStateMustResolveToSignalObject=off  FilterRTWStateStorageClass=Auto  ParallelPVariant=ExternalParameters  IdealPVariant=Disabled  IVariant=ExternalParameters  DVariant=Disabled  IntegratorVariant=Discrete  SatVariant=Enabled  AWVariant=DiscClampingParallel  PCopyVariant=Disabled  TRVariant=Disabled  FdbkBlocksVariant=Forward  IdealPFdbkVariant=Disabled  SatFdbkVariant=Disabled  DerivativeFilterVariant=Disabled  NVariant=Disabled  NCopyVariant=Disabled_SignalSpec  FilterICVariant=Disabled  IntegratorICVariant=ExternalICs  ExternalResetVariant=ExternalReset  TRSumVariant=Passthrough  SumFdbkVariant=Disabled  SumVariant=Sum_PI  TsampFilterVariant=InternalTs  TsampNgainVariant=Passthrough  TsampIntegralVariant=Passthrough  ExternalSaturationOutDataTypeStr=Inherit: Same as second input  aMode=5
  Ki : Constant  Value=PI_params.Ki_i*Ts/2  OutDataTypeStr=dataType  SampleTime=-1
  Kp : Constant  Value=PI_params.Kp_i/2  OutDataTypeStr=dataType2  SampleTime=-1
  Kp1 : Constant  Value=0  OutDataTypeStr=dataType  SampleTime=-1
  Logical Operator : Logic  Operator=NOT  IconShape=distinctive  AllPortsSameDT=off  OutDataTypeStr=boolean
  Sum : Sum  Inputs=|+-  OutDataTypeStr=Inherit: Same as first input
  V_ref : Outport  VectorParamsAs1DForOutWhenUnconnected=off
  wires:
  Discrete PI Controller with anti-windup & reset/1 -> V_ref/1
  Data Store Read1/1 -> AND/1
  I_fb/1 -> Sum/2
  I_ref/1 -> Sum/1
  Kp/1 -> Discrete PI Controller with anti-windup & reset/2
  Sum/1 -> Discrete PI Controller with anti-windup & reset/1
  Ki/1 -> Discrete PI Controller with anti-windup & reset/3
  Logical Operator/1 -> Discrete PI Controller with anti-windup & reset/4
  Kp1/1 -> Discrete PI Controller with anti-windup & reset/5
  Data Store Read/1 -> AND/2
  AND/1 -> Logical Operator/1

== system dsPIC33CK256MP508_MCLV2_QEI_Generator/Hardware Init/Enable Switch/Codegen ==
  note: Toggle between enable and disable on press on Button S2
  Button S2 : MCHP_Blockset/Digital IO/Digital Input  PORT=Dynamic Options  PORT_TXT="D   [ 0 : 15 ]"  PIN=5  PACK=off  SIMULTANEOUS=off  ORDERING=None  SampleTime=-1  MCHP_PORT={Digital In}{DIN}2:0:D5;  MCHP_MASTERLINK=dsPIC33CK256MP508_MCLV2_QEI_Generator/Hardware Init/Microchip Master
      settings: SourceProductName=MPLAB Device Blocks for Simulink
  Triggered Subsystem : Subsystem  TreatAsAtomicUnit=on
  wires:
  Button S2/1 -> Triggered Subsystem/Trigger

== system dsPIC33CK256MP508_MCLV2_QEI_Generator/Hardware Init/Enable Switch/Sim ==
  Constant : Constant  OutDataTypeStr=Inherit: Inherit via back propagation
  Data Store Write : DataStoreWrite  DataStoreName=Enable  IndexOptions=Index vector (dialog)  Indices=1  OutputSizes=1
  wires:
  Constant/1 -> Data Store Write/1

== system dsPIC33CK256MP508_MCLV2_QEI_Generator/Input Scaling/Quadrature Decoder/PositionNoReset ==
  Index : Inport
  Count : Inport  Port=2
  Action Port : ActionPort  ActionPortLabel=if(u1 > 0)
  CountsPerRevolution : Constant  Value=EncoderSlitsPerRevolution*1  OutDataTypeStr=Inherit: Inherit via back propagation
  MinMax : MinMax  Inputs=2  RndMeth=Simplest  ZeroCross=off
  Sum3 : Sum  Inputs=+-|  OutDataTypeStr=Inherit: Same as accumulator  RndMeth=Simplest
  Sum7 : Sum  Inputs=|++  OutDataTypeStr=Inherit: Same as accumulator  RndMeth=Simplest
  Position : Outport  VectorParamsAs1DForOutWhenUnconnected=off
  wires:
  Index/1 -> Sum3/2
  Count/1 -> Sum3/1
  Sum7/1 -> MinMax/2
  CountsPerRevolution/1 -> Sum7/2
  Sum3/1 -> Sum7/1, MinMax/1
  MinMax/1 -> Position/1

== system dsPIC33CK256MP508_MCLV2_QEI_Generator/Input Scaling/Quadrature Decoder/PositionResetAtIndex ==
  Count : Inport
  Action Port : ActionPort  ActionPortLabel=else
  Position : Outport  VectorParamsAs1DForOutWhenUnconnected=off
  wires:
  Count/1 -> Position/1

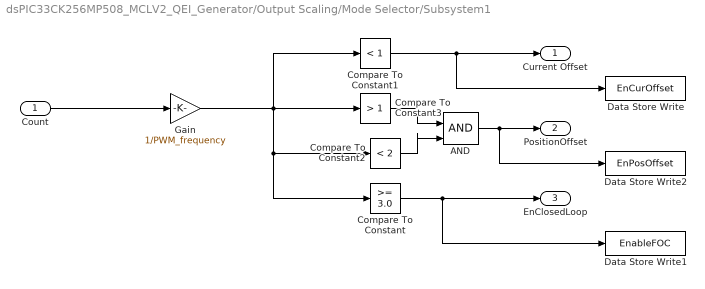
== system dsPIC33CK256MP508_MCLV2_QEI_Generator/Output Scaling/Mode Selector/Subsystem1 ==
  Count : Inport
  AND : Logic  IconShape=distinctive  AllPortsSameDT=off  OutDataTypeStr=boolean
  Compare To Constant : simulink/Logic and Bit Operations/Compare To Constant  relop=>=  const=3.0  OutDataTypeStr=boolean
  Compare To Constant1 : simulink/Logic and Bit Operations/Compare To Constant  relop=<  const=1  OutDataTypeStr=boolean
  Compare To Constant2 : simulink/Logic and Bit Operations/Compare To Constant  relop=<  const=2  OutDataTypeStr=boolean
  Compare To Constant3 : simulink/Logic and Bit Operations/Compare To Constant  relop=>  const=1  OutDataTypeStr=boolean
  Data Store Write : DataStoreWrite  DataStoreName=EnCurOffset  IndexOptions=Index vector (dialog)  Indices=1  OutputSizes=1
  Data Store Write1 : DataStoreWrite  DataStoreName=EnableFOC  IndexOptions=Index vector (dialog)  Indices=1  OutputSizes=1
  Data Store Write2 : DataStoreWrite  DataStoreName=EnPosOffset  IndexOptions=Index vector (dialog)  Indices=1  OutputSizes=1
  Gain : Gain  Gain=1/PWM_frequency  OutDataTypeStr=dataType2  RndMeth=Simplest
  Current Offset : Outport
  PositionOffset : Outport  Port=2
  EnClosedLoop : Outport  Port=3
  wires:
  Count/1 -> Gain/1
  Gain/1 -> Compare To Constant1/1, Compare To Constant3/1, Compare To Constant2/1, Compare To Constant/1
  Compare To Constant/1 -> Data Store Write1/1, EnClosedLoop/1
  Compare To Constant1/1 -> Data Store Write/1, Current Offset/1
  Compare To Constant2/1 -> AND/2
  Compare To Constant3/1 -> AND/1
  AND/1 -> Data Store Write2/1, PositionOffset/1

== system dsPIC33CK256MP508_MCLV2_QEI_Generator/Output Scaling/Mode Selector/Up Counter ==
  Enable : EnablePort  StatesWhenEnabling=reset
  Add1 : Sum  SaturateOnIntegerOverflow=on
  Constant : Constant  OutDataTypeStr=uint32
  Delay : Delay  DelayLength=1
  Count : Outport  InitialOutput=0
  wires:
  Delay/1 -> Add1/2
  Add1/1 -> Count/1, Delay/1
  Constant/1 -> Add1/1

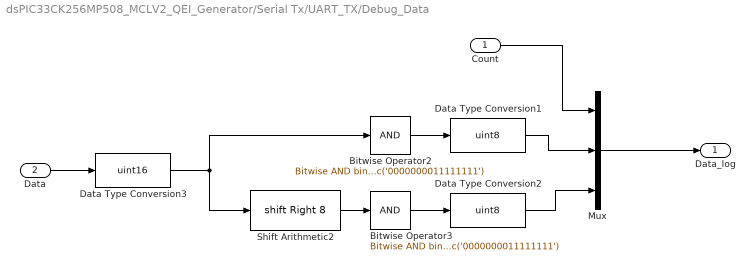
== system dsPIC33CK256MP508_MCLV2_QEI_Generator/Serial Tx/UART_TX/Debug_Data ==
  Count : Inport
  Data : Inport  Port=2
  Bitwise Operator2 : simulink/Logic and Bit Operations/Bitwise Operator  logicop=AND  UseBitMask=on  BitMask=bin2dec('0000000011111111')  BitMaskRealWorld=Stored Integer
  Bitwise Operator3 : simulink/Logic and Bit Operations/Bitwise Operator  logicop=AND  UseBitMask=on  BitMask=bin2dec('0000000011111111')  BitMaskRealWorld=Stored Integer
  Data Type Conversion1 : DataTypeConversion  OutDataTypeStr=uint8  RndMeth=Simplest  SaturateOnIntegerOverflow=off
  Data Type Conversion2 : DataTypeConversion  OutDataTypeStr=uint8  RndMeth=Simplest  SaturateOnIntegerOverflow=off
  Data Type Conversion3 : DataTypeConversion  OutDataTypeStr=uint16  ConvertRealWorld=Stored Integer (SI)  RndMeth=Simplest  SaturateOnIntegerOverflow=off
  Mux : Mux  Inputs=3
  Shift Arithmetic2 : ArithShift  BitShiftNumber=8  BitShiftDirection=Right
  Data_log : Outport
  wires:
  Mux/1 -> Data_log/1
  Data/1 -> Data Type Conversion3/1
  Count/1 -> Mux/1
  Bitwise Operator2/1 -> Data Type Conversion1/1
  Shift Arithmetic2/1 -> Bitwise Operator3/1
  Bitwise Operator3/1 -> Data Type Conversion2/1
  Data Type Conversion3/1 -> Bitwise Operator2/1, Shift Arithmetic2/1
  Data Type Conversion1/1 -> Mux/2
  Data Type Conversion2/1 -> Mux/3

== system dsPIC33CK256MP508_MCLV2_QEI_Generator/Serial Tx/UART_TX/SCI_Tx ==
  Data_Log : Inport
  End : Constant  Value=hex2dec('45')  OutDataTypeStr=uint8
  Mux : Mux  Inputs=3
  Start : Constant  Value=hex2dec('53')  OutDataTypeStr=uint8
  UART Tx : MCHP_Blockset/BUS UART/UART Tx  UART_REF=2  ORDERING=None  AllOrNothing=off  SampleTime=-1  MCHP_MASTERLINK=dsPIC33CK256MP508_MCLV2_QEI_Generator/Hardware Init/Microchip Master  NSend_Input=off  UART_String=off  NSend_Output=off
      settings: SourceProductName=MPLAB Device Blocks for Simulink
  wires:
  Mux/1 -> UART Tx/1
  Data_Log/1 -> Mux/2
  Start/1 -> Mux/1
  End/1 -> Mux/3

== system dsPIC33CK256MP508_MCLV2_QEI_Generator/Hardware Init/Enable Switch/Codegen/Triggered Subsystem ==
  Trigger : TriggerPort  TriggerType=falling  VariantControl=Variant
  Data Store Write : DataStoreWrite  DataStoreName=Enable  IndexOptions=Index vector (dialog)  Indices=1  OutputSizes=1
  Delay : Delay  DelayLength=1  InitialCondition=0
  NOT : Logic  Operator=NOT  IconShape=distinctive  AllPortsSameDT=off  OutDataTypeStr=boolean
  wires:
  NOT/1 -> Data Store Write/1, Delay/1
  Delay/1 -> NOT/1
